simulink model "tire_model"  (R2020a)
settings: Solver=VariableStepAuto  StartTime=0.0  StopTime=10.0  RelTol=1e-3
PostLoadFcn:
  | [Cstruct_lat]=load('pacejka_coefficients_lateral.mat');
  | Coeff_lat=Cstruct_lat.C;
  | [Cstruct_long]=load('pacejka_coefficients_longitudinal.mat');
  | Coeff_long=Cstruct_long.C;
settings Model: DataDictionary=Properties.sldd  Creator=yafta  LastModifiedBy=yafta

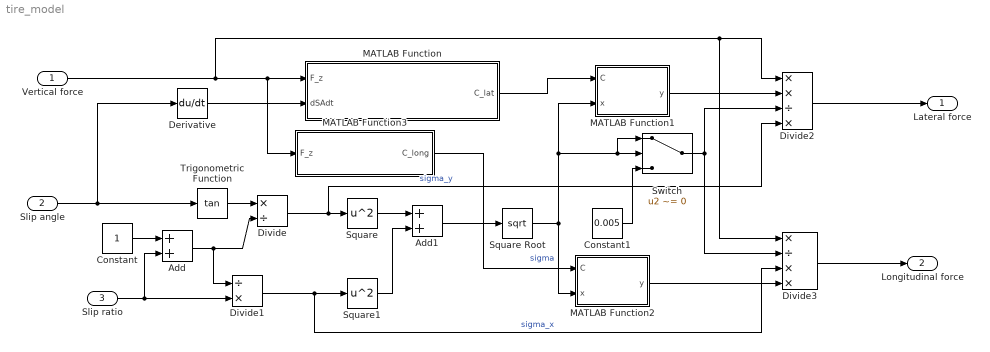
== system tire_model ==
  Vertical force : Inport  OutDataTypeStr=double
  Slip angle : Inport  Port=2  OutDataTypeStr=double
  Slip ratio : Inport  Port=3  OutDataTypeStr=double
  Add : Sum  Inputs=2
  Add1 : Sum
  Constant : Constant  OutDataTypeStr=double
  Constant1 : Constant  Value=0.005
  Derivative : Derivative
  Divide : Product  Inputs=*/
  Divide1 : Product  Inputs=/*
  Divide2 : Product  Inputs=**/*
  Divide3 : Product  Inputs=*/**
  MATLAB Function : MATLAB Function  TreatAsAtomicUnit=on
  MATLAB Function1 : MATLAB Function  TreatAsAtomicUnit=on
  MATLAB Function2 : MATLAB Function  TreatAsAtomicUnit=on
  MATLAB Function3 : MATLAB Function  TreatAsAtomicUnit=on
  Square : Math  Operator=square  SaturateOnIntegerOverflow=on
  Square Root : Sqrt  SaturateOnIntegerOverflow=on
  Square1 : Math  Operator=square  SaturateOnIntegerOverflow=on
  Switch : Switch  Criteria=u2 ~= 0
  Trigonometric Function : Trigonometry  Operator=tan  OutputSignalType=real
  Lateral force : Outport  OutDataTypeStr=double
  Longitudinal force : Outport  Port=2  OutDataTypeStr=double
  wires:
  Square Root/1 -> MATLAB Function1/2(x), Switch/1, Switch/2, MATLAB Function2/2(x)  "sigma"
  MATLAB Function3/1(C_long) -> MATLAB Function2/1(C)
  Vertical force/1 -> MATLAB Function3/1(F_z), MATLAB Function/1(F_z), Divide2/1, Divide3/1
  Divide1/1 -> Square1/1, Divide3/3  "sigma_x"
  Constant/1 -> Add/1
  Add/1 -> Divide/2, Divide1/1
  MATLAB Function2/1(y) -> Divide3/4
  Divide3/1 -> Longitudinal force/1
  Add1/1 -> Square Root/1
  Trigonometric Function/1 -> Divide/1
  Square1/1 -> Add1/2
  Derivative/1 -> MATLAB Function/2(dSAdt)
  Divide2/1 -> Lateral force/1
  Slip angle/1 -> Derivative/1, Trigonometric Function/1
  Square/1 -> Add1/1
  Divide/1 -> Square/1, Divide2/4  "sigma_y"
  MATLAB Function/1(C_lat) -> MATLAB Function1/1(C)
  MATLAB Function1/1(y) -> Divide2/2
  Slip ratio/1 -> Divide1/2, Add/2
  Constant1/1 -> Switch/3
  Switch/1 -> Divide3/2, Divide2/3

== matlab function tire_model/MATLAB Function ==
  data: F_z input; dSAdt input; C_lat output
function C_lat  = find_lat_coefficients(F_z,dSAdt)
n=0;
if F_z < -970
    n=1;
elseif F_z < -760
    n=3;
elseif F_z < -550
    n=5;
elseif F_z < -340
    n=7;
else
    n=5;
end
if dSAdt >= 0
    n=n+1;
end
%C_lat=Coeff_lat(n,:);
C_lat=[7.8048,2.5045,1.4395,0.4852];
end

== matlab function tire_model/MATLAB Function2 ==
  data: C input; y output; x input
function y = pacejka(C,x)
y=C(3)*sin(C(2)*atan(C(1)*(1-C(4))*x+C(4)*atan(C(1)*x)));
end

== matlab function tire_model/MATLAB Function3 ==
  data: F_z input; C_long output
function C_long = find_long_coefficients(F_z)
n=0;
if F_z < -960
    n=1;
elseif F_z < -760
    n=2;
elseif F_z < -400
    n=3;
else
    n=5;
end
%C_long=Coeff_long(1,:);
C_long=[-1.1829,-23.7950,-1.4949,98.0342];
end

== matlab function tire_model/MATLAB Function1 ==
  data: C input; y output; x input
function y = pacejka(C,x)
y=C(3)*sin(C(2)*atan(C(1)*(1-C(4))*x+C(4)*atan(C(1)*x)));
end
